simulink model "HvCoorn"  (R2022b)
settings: configuration reference "Icar05FusaMdlCfg" (kept outside this file)
undefined symbols (not defined in the file): BMSActSt_ACChrg, BMSActSt_DCChrg, BMSActSt_disconnect, BMSActSt_offline, BMSActSt_online, BMSActSt_undefined, BMSMainNegRlySt_Clsd_SC, BMSMainNegRlySt_Open_SC, BMSMainNegRlySt_StuckInClsd_SC, BMSMainNegRlySt_StuckInOpen_SC, BMSMainPosRlySt_Clsd_SC, BMSMainPosRlySt_Open_SC, BMSMainPosRlySt_StuckInClsd_SC, BMSPrecRlySt_StuckInOpen_SC, BMSReqSt_ACChrg, BMSReqSt_DCChrg, BMSReqSt_emergencyOffline, BMSReqSt_offline, BMSReqSt_online, Chrg_stCycleBookMod_SC, Chrg_stSingleBookMod_SC, CmpgMod_stInactv_SC, DCDCActSt_buck, DCDCActSt_connected, DCDCActSt_disconnected, DCDCReqSt_buck, DCDCReqSt_standby, EngStrtStop_RefuModDft_SC, EPBActSt_Appld_SC, GearLvr_stDrvGearD_SC, GearLvr_stDrvGearN_SC, GearLvr_stDrvGearP_SC, GearLvr_stDrvGearR_SC, hpp_bACChargeLinkIni_C, hpp_bACChargeLinkOKIni_C, hpp_bAcChgEnaIni_C, hpp_bAcChgPauseIni_C, hpp_bAcLinkTempErrIni_C, hpp_bBattWarmReqIni_C, hpp_bHvilHwErrIni_C, hpp_bHvilStOkIni_C, hpp_bHvRelayClsActIni_C, hpp_bHvRelayOpnActIni_C, hpp_bHvRelayStuckIni_C, hpp_bParked4ChDchgIni_C, hpp_bRemLvBatMntnReqIni_C, hpp_bStartUpReqIni_C, hpp_stHvilCanIni_C, hpp_stWarmTimeCfgRespIni_C, HvCoorn_bAuthEnaSwt_C, HvCoorn_bAuthFailSpdLimOvrd_C, HvCoorn_bAuthFailSpdLimOvrdVal_C, HvCoorn_bAuthStrt_C, HvCoorn_bBMSUnexpdDcnctFailEna_C, HvCoorn_bBuck2RdyBypDCDCEna_C, HvCoorn_bDCChrgFctCfg_C, HvCoorn_bDcChrgWkupEnaChrgLink_C, HvCoorn_bDCDcnct4ACEna_C, HvCoorn_bDCNotBuck2ShtdwnEna_C, HvCoorn_bDrvrLevNotRdyEna_C ... (+295)
libraries: ITKLib x213, simulink x61
(part 8 of 12)

== system HvCoorn/HvCoorn/HVP_HighVoltagePowerOnOffProcedure/A29_V2In ==
  idi_bKeyOn : Inport
  HvCoorn_stHVP : Inport  Port=2
  PwrLimBatt_pwrContnsDChrg : Inport  Port=3
  icbms_pctHVBatSOCDisp : Inport  Port=4
  icobc_stOBCModeV2In : Inport  Port=5
  icobc_stChrgrCnct : Inport  Port=6
  icicm_stIvtrEnaSwt : Inport  Port=7
  ibsw_bCnctElecDvce : Inport  Port=8
  ved_bHvShtdwn : Inport  Port=9
  icobc_stOBCMode : Inport  Port=10
  icobc_stV2LFltTyp : Inport  Port=11
  icicm_bOTAOn : Inport  Port=12
  AND : Logic  Inputs=7  OutDataTypeStr=boolean
  AND1 : Logic  Operator=OR  Inputs=9  OutDataTypeStr=boolean
  AND2 : Logic  OutDataTypeStr=boolean
  AND3 : Logic  OutDataTypeStr=boolean
  AND4 : Logic  OutDataTypeStr=boolean
  AND6 : Logic  Operator=OR  OutDataTypeStr=boolean
  Calibration1 : Constant  Description=[3300]  Value=HvCoorn_pwrBattV2InEnaLowLim_C  SampleTime=-1
      settings: AttributesFormatString=%<Description>
  Calibration2 : Constant  Description=[3300]  Value=HvCoorn_pwrBattV2InExHighLim_C  SampleTime=-1
      settings: AttributesFormatString=%<Description>
  Calibration3 : Constant  Description=[3600]  Value=HvCoorn_tiDiscnctDvceExThd_C  SampleTime=-1
      settings: AttributesFormatString=%<Description>
  Calibration4 : Constant  Description=[1]  Value=HvCoorn_bOTAOnExV2InEna_C  SampleTime=-1
      settings: AttributesFormatString=%<Description>
  Constant10 : Constant  Description=[1]  Value=OBCChrgrCnctnSt_Cnct_SC
      settings: AttributesFormatString=%<Description>
  Constant2 : Constant  Description=[8]  Value=OBCActSt_V2In
      settings: AttributesFormatString=[8]
  Constant3 : Constant  Description=[4]  Value=OBCActSt_V2LAndV2In
      settings: AttributesFormatString=[4]
  Constant4 : Constant  Description=[7]  Value=OBCActSt_failure
      settings: AttributesFormatString=[7]
  Constant5 : Constant  Description=[3]  Value=OBCActSt_charging
      settings: AttributesFormatString=[3]
  Constant6 : Constant  Description=[7]  Value=OBCActSt_failure
      settings: AttributesFormatString=[7]
  Constant9 : Constant  Description=[0]  Value=OBCChrgrCnctnSt_Dcnct_SC
      settings: AttributesFormatString=%<Description>
  EdgeFalling : ITKLib/Memory/EdgeFalling  Tag=initial value = 0
      settings: SourceProductName=ITKC_Lib
  EdgeFalling1 : ITKLib/Memory/EdgeFalling  Tag=initial value = 0
      settings: SourceProductName=ITKC_Lib
  EdgeRising : ITKLib/Memory/EdgeRising  Tag=initial value = 0
      settings: SourceProductName=ITKC_Lib
  Equal{,1,6..11,13..15,17} (12 alike) : RelationalOperator  Operator===  OutDataTypeStr=boolean  RndMeth=Simplest  InputSameDT=off
  Equal12 : RelationalOperator  Operator=<  OutDataTypeStr=boolean  RndMeth=Simplest  InputSameDT=off
  Equal16 : RelationalOperator  Operator=<  OutDataTypeStr=boolean  RndMeth=Simplest  InputSameDT=off
  Equal2 : RelationalOperator  OutDataTypeStr=boolean  RndMeth=Simplest  InputSameDT=off
  Equal3 : RelationalOperator  Operator=>  OutDataTypeStr=boolean  RndMeth=Simplest  InputSameDT=off
  Equal4 : RelationalOperator  Operator=~=  OutDataTypeStr=boolean  RndMeth=Simplest  InputSameDT=off
  Equal5 : RelationalOperator  Operator=~=  OutDataTypeStr=boolean  RndMeth=Simplest  InputSameDT=off
  Not1 : Logic  Operator=NOT  AllPortsSameDT=off  OutDataTypeStr=boolean
  Not6 : Logic  Operator=NOT  AllPortsSameDT=off  OutDataTypeStr=boolean
  OR : Logic  Operator=OR  OutDataTypeStr=boolean
  OR1 : Logic  Operator=OR  OutDataTypeStr=boolean
  OR2 : Logic  Operator=OR  Inputs=3  OutDataTypeStr=boolean
  OR3 : Logic  Operator=OR  Inputs=3  OutDataTypeStr=boolean
  OR7 : Logic  OutDataTypeStr=boolean
  OR8 : Logic  OutDataTypeStr=boolean
  RSLatch : ITKLib/Memory/RSLatch
      settings: SourceProductName=ITKC_Lib
  RSLatch1 : ITKLib/Memory/RSLatch
      settings: SourceProductName=ITKC_Lib
  TaskTime_s2 : Constant  Value=TaskTime_10ms
      settings: AttributesFormatString=[0.01]
  Terminator : Terminator
  TurnOnDelayVari : ITKLib/TimeCounter/TurnOnDelayVari
      settings: AttributesFormatString=TurnOnDelay  SourceProductName=ITKC_Lib
  UnitDelay : UnitDelay  SampleTime=-1  HasFrameUpgradeWarning=on
      settings: AttributesFormatString=<Initial=%<x0>>
  hpp_tiRemHvBatPrecdngSet_C1 : Constant  Description=[20]  Value=HvCoorn_pctHvBatSocV2InExThd_C
      settings: AttributesFormatString=%<Description>
  hpp_tiRemHvBatPrecdngSet_C2 : Constant  Description=[20]  Value=HvCoorn_pctHvBatSocV2InActvThd_C
      settings: AttributesFormatString=%<Description>
  uint1 : Constant  Value=90  OutDataTypeStr=uint8  SampleTime=-1
      settings: AttributesFormatString=%<OutDataTypeStr>
  uint10 : Constant  Value=2  OutDataTypeStr=uint8  SampleTime=-1
      settings: AttributesFormatString=%<OutDataTypeStr>
  uint11 : Constant  Value=3  OutDataTypeStr=uint8  SampleTime=-1
      settings: AttributesFormatString=%<OutDataTypeStr>
  uint2 : Constant  Value=2  OutDataTypeStr=uint8  SampleTime=-1
      settings: AttributesFormatString=%<OutDataTypeStr>
  uint4 : Constant  OutDataTypeStr=uint8  SampleTime=-1
      settings: AttributesFormatString=%<OutDataTypeStr>
  uint8 : Constant  Value=89  OutDataTypeStr=uint8  SampleTime=-1
      settings: AttributesFormatString=%<OutDataTypeStr>
  uint9 : Constant  OutDataTypeStr=uint8  SampleTime=-1
      settings: AttributesFormatString=%<OutDataTypeStr>
  HvCoorn_bV2InReq : Outport  VectorParamsAs1DForOutWhenUnconnected=off
  HvCoorn_bV2InEna : Outport  Port=2  VectorParamsAs1DForOutWhenUnconnected=off
  wires:
  uint8/1 -> Equal/2
  HvCoorn_stHVP/1 -> Equal1/1, Equal/1
  uint1/1 -> Equal1/2
  Equal/1 -> OR/1
  Equal1/1 -> OR/2
  PwrLimBatt_pwrContnsDChrg/1 -> Equal2/1, [PwrLimBatt_pwrContnsDChrg]
  Calibration1/1 -> Equal2/2
  icbms_pctHVBatSOCDisp/1 -> Equal3/1, [icbms_pctHVBatSOCDisp]
  hpp_tiRemHvBatPrecdngSet_C2/1 -> Equal3/2
  [icobc_stOBCMode] -> Equal5/1, Equal4/1
  icobc_stChrgrCnct/1 -> Equal6/1, [icobc_stChrgrCnct]
  Constant9/1 -> Equal6/2
  uint2/1 -> Equal7/2  "Enable"
  icicm_stIvtrEnaSwt/1 -> Equal13/1, Equal7/1
  Equal7/1 -> OR1/1
  ibsw_bCnctElecDvce/1 -> [ibsw_bCnctElecDvce], EdgeRising/1, EdgeFalling1/1, Not1/1
  Equal2/1 -> AND/3
  Equal3/1 -> AND/4
  OR/1 -> AND/1
  idi_bKeyOn/1 -> [idi_bKeyOn], AND/2
  AND/1 -> RSLatch/1  "HvCoorn_bV2InEnaRawSet"
  icobc_stOBCMode/1 -> [icobc_stOBCMode], Equal9/1
  Constant4/1 -> Equal9/2
  [icobc_stChrgrCnct] -> Equal10/1
  Constant10/1 -> Equal10/2
  Calibration2/1 -> Equal12/2
  [PwrLimBatt_pwrContnsDChrg] -> Equal12/1
  Equal12/1 -> AND1/7
  Equal10/1 -> AND1/5
  Equal9/1 -> AND1/4
  Equal16/1 -> AND1/3
  ved_bHvShtdwn/1 -> AND1/2
  OR3/1 -> AND1/1
  uint4/1 -> Equal13/2  "Disable"
  Equal13/1 -> OR3/1
  AND1/1 -> RSLatch/2  "HvCoorn_bV2InEnaRawRst"
  RSLatch/1 -> UnitDelay/1, HvCoorn_bV2InReq/1, OR7/1
  Constant2/1 -> Equal17/2
  [icobc_stOBCMode] -> Equal17/1
  OR7/1 -> HvCoorn_bV2InEna/1
  Equal6/1 -> AND/6
  OR1/1 -> AND/7
  [icbms_pctHVBatSOCDisp] -> Equal16/1
  hpp_tiRemHvBatPrecdngSet_C1/1 -> Equal16/2
  [idi_bKeyOn] -> EdgeFalling/1
  EdgeFalling/1 -> AND1/6
  TaskTime_s2/1 -> TurnOnDelayVari/2
  Calibration3/1 -> TurnOnDelayVari/3
  TurnOnDelayVari/1 -> OR3/3
  Equal8/1 -> AND6/2
  [icobc_stOBCMode] -> Equal8/1
  Constant3/1 -> Equal8/2
  Equal17/1 -> AND6/1
  AND6/1 -> OR7/2
  OR8/1 -> AND/5
  icobc_stOBCModeV2In/1 -> Terminator/1
  Equal4/1 -> OR8/1
  Equal5/1 -> OR8/2
  Constant5/1 -> Equal4/2
  Constant6/1 -> Equal5/2
  EdgeRising/1 -> OR1/2
  UnitDelay/1 -> [HvCoorn_bV2InReqOld]
  Not1/1 -> AND2/1
  [HvCoorn_bV2InReqOld] -> AND2/2
  AND2/1 -> TurnOnDelayVari/1
  [HvCoorn_bV2InReqOld] -> AND3/2
  AND3/1 -> OR3/2
  EdgeFalling1/1 -> AND3/1
  uint10/1 -> Equal11/2
  icobc_stV2LFltTyp/1 -> Equal11/1, Equal14/1, Equal15/1
  uint9/1 -> Equal15/2
  uint11/1 -> Equal14/2
  [ibsw_bCnctElecDvce] -> Not6/1
  Not6/1 -> RSLatch1/2
  Equal14/1 -> OR2/3
  Equal11/1 -> OR2/2
  Equal15/1 -> OR2/1
  OR2/1 -> RSLatch1/1
  RSLatch1/1 -> AND1/9
  AND4/1 -> AND1/8
  icicm_bOTAOn/1 -> AND4/1
  Calibration4/1 -> AND4/2

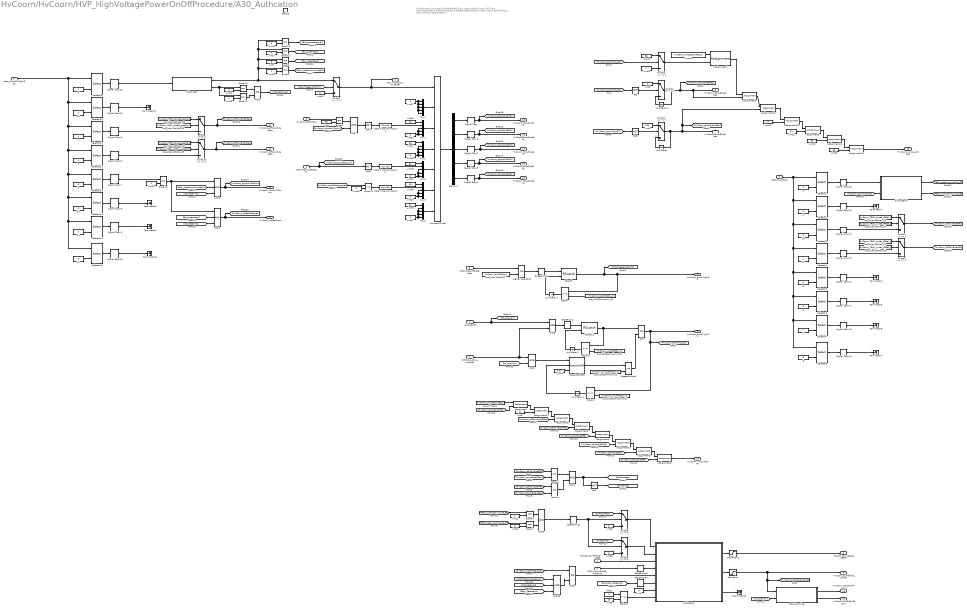
== system HvCoorn/HvCoorn/HVP_HighVoltagePowerOnOffProcedure/A30_Authcation ==
  note: 指令类型
      | 0000无效:0
      | 0001平台网络连接通讯丢失:1
      | 0010防盗校验:2
      | 0011密钥下发:3
      | 0100异常次数清除:4
      | 0101异常次数同步:5
      |
      | 接收模块
      | 0000全部ECU:0
      | 0001仅VCU:1
      | 0010仅BMS:2
      | 0011仅RMCU:3
      | 0100仅TBOX:4
  VCU_E2_counterfaieldEER : Inport
  idi_bKeyOn : Inport  Port=2
  VCCM_flg_Allow_Antitheft : Inport  Port=3
  VCCM_flg_Antitheft_Overtime : Inport  Port=4
  VCCM_flg_Antitheft_Start : Inport  Port=5
  ictcp_noAuthChlgOnReq : Inport  Port=6
  ictcp_noAuthSts : Inport  Port=7
  HvCoorn_stHVPOld : Inport  Port=8
  VCCM_flg_SK_Recep_ok : Inport  Port=9
  Enable : EnablePort
  1 : Constant  Value=3  OutDataTypeStr=single
  10 : Constant  Value=3  OutDataTypeStr=single
  11 : Constant  Value=4  OutDataTypeStr=single
  12 : Constant  Value=5  OutDataTypeStr=single
  13 : Constant  Value=6  OutDataTypeStr=single
  14 : Constant  Value=7  OutDataTypeStr=single
  15 : Constant  Value=8  OutDataTypeStr=single
  16 : Constant  Value=2  OutDataTypeStr=single
  2 : Constant  Value=4  OutDataTypeStr=single
  3 : Constant  Value=5  OutDataTypeStr=single
  4 : Constant  OutDataTypeStr=single
  5 : Constant  OutDataTypeStr=single
  6 : Constant  Value=6  OutDataTypeStr=single
  7 : Constant  Value=7  OutDataTypeStr=single
  8 : Constant  Value=8  OutDataTypeStr=single
  9 : Constant  Value=2  OutDataTypeStr=single
  AND{1,5..8} (5 alike) : Logic  OutDataTypeStr=boolean
  AND10 : Logic  Inputs=3  OutDataTypeStr=boolean
  AND2 : Logic  Operator=OR  OutDataTypeStr=boolean
  AND3 : Logic  Inputs=3  OutDataTypeStr=boolean
  AND4 : Logic  Inputs=3  OutDataTypeStr=boolean
  AND9 : Logic  Operator=OR  OutDataTypeStr=boolean
  Assignment : Assignment  DiagnosticForDimensions=Warning  IndexOptions=Index vector (dialog)  Indices=1  OutputSizes=1
  Assignment1 : Assignment  DiagnosticForDimensions=Warning  IndexOptions=Index vector (dialog)  Indices=6  OutputSizes=1
  Assignment10 : Assignment  DiagnosticForDimensions=Warning  IndexOptions=Index vector (dialog)  Indices=4  OutputSizes=1
  Assignment11 : Assignment  DiagnosticForDimensions=Warning  IndexOptions=Index vector (dialog)  Indices=5  OutputSizes=1
  Assignment12 : Assignment  DiagnosticForDimensions=Warning  IndexOptions=Index vector (dialog)  Indices=7  OutputSizes=1
  Assignment13 : Assignment  DiagnosticForDimensions=Warning  IndexOptions=Index vector (dialog)  Indices=8  OutputSizes=1
  Assignment14 : Assignment  DiagnosticForDimensions=Warning  IndexOptions=Index vector (dialog)  Indices=2  OutputSizes=1
  Assignment2 : Assignment  DiagnosticForDimensions=Warning  IndexOptions=Index vector (dialog)  Indices=3  OutputSizes=1
  Assignment3 : Assignment  DiagnosticForDimensions=Warning  IndexOptions=Index vector (dialog)  Indices=4  OutputSizes=1
  Assignment4 : Assignment  DiagnosticForDimensions=Warning  IndexOptions=Index vector (dialog)  Indices=5  OutputSizes=1
  Assignment5 : Assignment  DiagnosticForDimensions=Warning  IndexOptions=Index vector (dialog)  Indices=7  OutputSizes=1
  Assignment6 : Assignment  DiagnosticForDimensions=Warning  IndexOptions=Index vector (dialog)  Indices=8  OutputSizes=1
  Assignment7 : Assignment  DiagnosticForDimensions=Warning  IndexOptions=Index vector (dialog)  Indices=1  OutputSizes=1
  Assignment8 : Assignment  DiagnosticForDimensions=Warning  IndexOptions=Index vector (dialog)  Indices=6  OutputSizes=1
  Assignment9 : Assignment  DiagnosticForDimensions=Warning  IndexOptions=Index vector (dialog)  Indices=3  OutputSizes=1
  Auth_status : Stateflow chart  TreatAsAtomicUnit=on
  B01_Warnning : Subsystem
  Data Type Conversion : DataTypeConversion  SaturateOnIntegerOverflow=off  RndMeth=Floor
  Data Type Conversion1 : DataTypeConversion  SaturateOnIntegerOverflow=off  RndMeth=Floor
  Data Type Conversion2 : DataTypeConversion  SaturateOnIntegerOverflow=off  RndMeth=Floor
  Delay : Delay  DelayLengthSource=Input port  DelayLengthUpperLimit=200
      settings: InputPortMap=u0,p1
  Delay1 : Delay  DelayLengthSource=Input port  DelayLengthUpperLimit=200
      settings: InputPortMap=u0,p1
  Delay2 : Delay  DelayLengthSource=Input port  DelayLengthUpperLimit=200
      settings: InputPortMap=u0,p1
  Delay3 : Delay  DelayLengthSource=Input port
      settings: InputPortMap=u0,p1
  Demux1 : Demux  Outputs=5
  EdgeRising{,1..4} (5 alike) : ITKLib/Memory/EdgeRising  Tag=initial value = 0
      settings: SourceProductName=ITKC_Lib
  Equal{1..2,6..8,10..13,15} (10 alike) : RelationalOperator  Operator===  OutDataTypeStr=boolean  RndMeth=Simplest  InputSameDT=off
  Equal14 : RelationalOperator  Operator=~=  OutDataTypeStr=boolean  RndMeth=Simplest  InputSameDT=off
  Equal3 : RelationalOperator  Operator===  OutDataTypeStr=boolean
  Equal4 : RelationalOperator  Operator===  OutDataTypeStr=boolean
  GreaterOrEqual : RelationalOperator  OutDataTypeStr=boolean
  Logical Operator6 : Logic  Operator=OR  AllPortsSameDT=off  OutDataTypeStr=boolean
  Multiport Switch : MultiPortSwitch  DataPortOrder=Zero-based contiguous  Inputs=6  zeroidx=on  SaturateOnIntegerOverflow=off  InputSameDT=off
  Mux{1..6} (6 alike) : Mux  Inputs=5
  Not{1..5} (5 alike) : Logic  Operator=NOT  AllPortsSameDT=off  OutDataTypeStr=boolean
  OR2 : Logic  Operator=OR  OutDataTypeStr=boolean
  RSLatch : ITKLib/Memory/RSLatch
      settings: SourceProductName=ITKC_Lib
  RSLatch1 : ITKLib/Memory/RSLatch
      settings: SourceProductName=ITKC_Lib
  Saturation : Saturate  UpperLimit=15  LowerLimit=0
  Saturation1 : Saturate  UpperLimit=15  LowerLimit=0
  Selector{1..16} (16 alike) : Selector  NumberOfDimensions=2  InputPortWidth=10  IndexOptions=Index vector (dialog),Index vector (port)  Indices=1,2  OutputSizes=1,1
  Signal Copy{,1..20} (21 alike) : SignalConversion  OverrideOpt=off
  StopWatchRE1 : ITKLib/TimeCounter/StopWatchRE  Description=""
      settings: SourceProductName=ITKC_Lib
  Subsystem : Subsystem
  Subsystem1 : Subsystem
  Switch{1..4,7..10} (8 alike) : Switch  Criteria=u2 ~= 0  SaturateOnIntegerOverflow=off  InputSameDT=off
      settings: AttributesFormatString=Criteria : %<Criteria>
  Switch5 : Switch  Criteria=u2 ~= 0  OutDataTypeStr=boolean  SaturateOnIntegerOverflow=off  InputSameDT=off
      settings: AttributesFormatString=Criteria : %<Criteria>
  Switch6 : Switch  Criteria=u2 ~= 0  OutDataTypeStr=boolean  SaturateOnIntegerOverflow=off  InputSameDT=off
      settings: AttributesFormatString=Criteria : %<Criteria>
  TRUE : Constant  Description=TRUE  OutDataTypeStr=boolean  SampleTime=-1
      settings: AttributesFormatString=%<Description>
  Terminator{1,4..10,12..13} (10 alike) : Terminator
  Unit Delay{,1..4} (5 alike) : UnitDelay  SampleTime=-1  HasFrameUpgradeWarning=on
      settings: AttributesFormatString=<initial=%<x0>>
  sup_bKeyStrtMan_C : Constant  Description=[0]  Value=HvCoorn_bAuthStrt_C
      settings: AttributesFormatString=%<Description>
  sup_bKeyStrtMan_C1 : Constant  Description=[0]  Value=HvCoorn_TBOX_byte4_FBSet_C
      settings: AttributesFormatString=%<Description>
  sup_bKeyStrtMan_C2 : Constant  Description=[0]  Value=HvCoorn_TBOX_byte4_FBCal_C
      settings: AttributesFormatString=%<Description>
  sup_bKeyStrtMan_C3 : Constant  Description=[0]  Value=HvCoorn_TBOX_byte5_FBCal_C
      settings: AttributesFormatString=%<Description>
  sup_bKeyStrtMan_C4 : Constant  Description=[0]  Value=HvCoorn_TBOX_byte5_FBSet_C
      settings: AttributesFormatString=%<Description>
  sup_bKeyStrtMan_C5 : Constant  Description=[0]  Value=HvCoorn_TBOX_byte5_reqCal_C
      settings: AttributesFormatString=%<Description>
  sup_bKeyStrtMan_C6 : Constant  Description=[0]  Value=HvCoorn_TBOX_byte5_reqSet_C
      settings: AttributesFormatString=%<Description>
  sup_bKeyStrtMan_C7 : Constant  Description=[0]  Value=HvCoorn_TBOX_byte4_reqCal_C
      settings: AttributesFormatString=%<Description>
  sup_bKeyStrtMan_C8 : Constant  Description=[0]  Value=HvCoorn_TBOX_byte4_reqSet_C
      settings: AttributesFormatString=%<Description>
  sup_tiChgConndown_C : Constant  Description=[1800]  Value=HvCoorn_tiAuthStartDly_C
      settings: AttributesFormatString=%<Description>
  sup_tiChgConndown_C1 : Constant  Description=[200]  Value=HvCoorn_nAuthRstDly_C
      settings: AttributesFormatString=%<Description>
  sup_tiChgConndown_C2 : Constant  Description=[200]  Value=HvCoorn_nAuthRstDly_C
      settings: AttributesFormatString=%<Description>
  sup_tiChgConndown_C3 : Constant  Description=[200]  Value=HvCoorn_nAuthRstDly_C
      settings: AttributesFormatString=%<Description>
  sup_uThres_C : Constant  Description="[0  0  0  0  0  0  0  0]"  Value=HvCoorn_uVCU2tboxFB_C  OutDataTypeStr=uint8
      settings: AttributesFormatString=%<Description>
  uint{1,15,24,29,31..35,37,40} (11 alike) : Constant  Value=0  OutDataTypeStr=uint8  SampleTime=-1
      settings: AttributesFormatString=%<OutDataTypeStr>
  uint{6,11,25..26,28} (5 alike) : Constant  OutDataTypeStr=uint8  SampleTime=-1
      settings: AttributesFormatString=%<OutDataTypeStr>
  uint12 : Constant  Value=2  OutDataTypeStr=uint8  SampleTime=-1
      settings: AttributesFormatString=%<OutDataTypeStr>
  uint13 : Constant  Value=17  OutDataTypeStr=uint8  SampleTime=-1
      settings: AttributesFormatString=%<OutDataTypeStr>
  uint2 : Constant  Value=17  OutDataTypeStr=uint8  SampleTime=-1
      settings: AttributesFormatString=%<OutDataTypeStr>
  uint21 : Constant  Value=34  OutDataTypeStr=uint8  SampleTime=-1
      settings: AttributesFormatString=%<OutDataTypeStr>
  uint22 : Constant  Value=51  OutDataTypeStr=uint8  SampleTime=-1
      settings: AttributesFormatString=%<OutDataTypeStr>
  uint23 : Constant  Value=68  OutDataTypeStr=uint8  SampleTime=-1
      settings: AttributesFormatString=%<OutDataTypeStr>
  uint27 : Constant  Value=4  OutDataTypeStr=uint8  SampleTime=-1
      settings: AttributesFormatString=%<OutDataTypeStr>
  uint3 : Constant  Value=100  OutDataTypeStr=uint8  SampleTime=-1
      settings: AttributesFormatString=%<OutDataTypeStr>
  uint36 : Constant  Value=20  OutDataTypeStr=uint8  SampleTime=-1
      settings: AttributesFormatString=%<OutDataTypeStr>
  uint38 : Constant  Value=0  OutDataTypeStr=boolean  SampleTime=-1
      settings: AttributesFormatString=%<OutDataTypeStr>
  uint39 : Constant  Value=0  OutDataTypeStr=boolean  SampleTime=-1
      settings: AttributesFormatString=%<OutDataTypeStr>
  uint4 : Constant  Description=SystemReadyWait  Value=89  OutDataTypeStr=uint8
      settings: AttributesFormatString=|
      | %<OutDataTypeStr>
      | %<Description>
  uint41 : Constant  Value=5  OutDataTypeStr=uint8  SampleTime=-1
      settings: AttributesFormatString=%<OutDataTypeStr>
  uint43 : Constant  Value=36  OutDataTypeStr=uint8  SampleTime=-1
      settings: AttributesFormatString=%<OutDataTypeStr>
  uint44 : Constant  Value=0.01  OutDataTypeStr=single  SampleTime=-1
      settings: AttributesFormatString=%<OutDataTypeStr>
  uint46 : Constant  Description="[0  0  0  0  0  0  0  0]"  Value=HvCoorn_uVCU2tboxReq_C  OutDataTypeStr=uint8  SampleTime=-1
      settings: AttributesFormatString=%<Description>
  uint47 : Constant  Value=36  OutDataTypeStr=uint8  SampleTime=-1
      settings: AttributesFormatString=%<OutDataTypeStr>
  uint48 : Constant  Value=52  OutDataTypeStr=uint8  SampleTime=-1
      settings: AttributesFormatString=%<OutDataTypeStr>
  uint49 : Constant  Value=68  OutDataTypeStr=uint8  SampleTime=-1
      settings: AttributesFormatString=%<OutDataTypeStr>
  uint5 : Constant  Value=10  OutDataTypeStr=uint8  SampleTime=-1
      settings: AttributesFormatString=%<OutDataTypeStr>
  uint50 : Constant  Value=84  OutDataTypeStr=uint8  SampleTime=-1
      settings: AttributesFormatString=%<OutDataTypeStr>
  uint7 : Constant  Value=3  OutDataTypeStr=uint8  SampleTime=-1
      settings: AttributesFormatString=%<OutDataTypeStr>
  VCU_Instruction_Type_FB : Outport  VectorParamsAs1DForOutWhenUnconnected=off
  HvCoorn_bAntiTrig430 : Outport  Port=2  VectorParamsAs1DForOutWhenUnconnected=off
  HvCoorn_bAntiTrig42C : Outport  Port=3  VectorParamsAs1DForOutWhenUnconnected=off
  VCU_E2_counterfaieldEEW : Outport  Port=4  VectorParamsAs1DForOutWhenUnconnected=off
  HvCoorn_authfailed_conter : Outport  Port=5  VectorParamsAs1DForOutWhenUnconnected=off
  HvCoorn_stVcuByte5Req : Outport  Port=6  VectorParamsAs1DForOutWhenUnconnected=off
  HvCoorn_stVcuByte4Req : Outport  Port=7  VectorParamsAs1DForOutWhenUnconnected=off
  HvCoorn_bAuthHvStrtLim : Outport  Port=8  VectorParamsAs1DForOutWhenUnconnected=off
  HvCoorn_bClearZero : Outport  Port=9  VectorParamsAs1DForOutWhenUnconnected=off
  HvCoorn_stAuthChkFailLvl : Outport  Port=10  VectorParamsAs1DForOutWhenUnconnected=off
  HvCoorn_stTboxByte5Req : Outport  Port=11  VectorParamsAs1DForOutWhenUnconnected=off
  HvCoorn_stTboxByte4Req : Outport  Port=12  VectorParamsAs1DForOutWhenUnconnected=off
  HvCoorn_stVcuByte3Fb : Outport  Port=13  VectorParamsAs1DForOutWhenUnconnected=off
  HvCoorn_stVcuByte2Fb : Outport  Port=14  VectorParamsAs1DForOutWhenUnconnected=off
  HvCoorn_stVcuByte1Fb : Outport  Port=15  VectorParamsAs1DForOutWhenUnconnected=off
  HvCoorn_stVcuByte0Fb : Outport  Port=16  VectorParamsAs1DForOutWhenUnconnected=off
  HvCoorn_noVcuAuthFb : Outport  Port=17  VectorParamsAs1DForOutWhenUnconnected=off
  HvCoorn_noVcuAuthReq : Outport  Port=18  VectorParamsAs1DForOutWhenUnconnected=off
  HvCoorn_stVcuByte7Fb : Outport  Port=19  VectorParamsAs1DForOutWhenUnconnected=off
  " HvCoorn_bAuthFailSpdLim" : Outport  Port=20  VectorParamsAs1DForOutWhenUnconnected=off
  wires:
  RSLatch/1 -> Delay/1, HvCoorn_bAntiTrig430/1, [VCU_Trigger_430_TX]
  [HvCoorn_bAntiTrig42C] -> Switch3/2
  uint43/1 -> Switch3/1
  uint15/1 -> Switch3/3
  Switch5/1 -> Auth_status/1(authsuccess)  "authsuccess"
  Saturation/1 -> HvCoorn_authfailed_conter/1, B01_Warnning/1(HvCoorn_authfailed_conter), [HvCoorn_authfailed_conter]  "HvCoorn_authfailed_conter"
  VCU_E2_counterfaieldEER/1 -> Auth_status/3(authfailed_n_conterEER)
  Auth_status/2(authfailed_n_conter) -> Saturation/1
  Auth_status/1(authfailed_n_conterEEW) -> Saturation1/1
  AND6/1 -> StopWatchRE1/1
  uint44/1 -> StopWatchRE1/3
  sup_tiChgConndown_C/1 -> GreaterOrEqual/2
  StopWatchRE1/1 -> GreaterOrEqual/1
  GreaterOrEqual/1 -> OR2/2
  Subsystem/2(TBOX_receiver_module_req) -> Equal10/1, Equal11/1
  Switch7/1 -> VCU_Instruction_Type_FB/1, Multiport Switch/1  "VCU_Instruction_Type_FB"
  [HvCoorn_stTboxByte5Fb] -> Equal3/1
  [HvCoorn_stTboxByte4Fb] -> Equal4/1
  AND1/1 -> [authsuccess], Not1/1
  Equal3/1 -> AND1/1
  [HvCoorn_stVcuByte5Req] -> Equal3/2
  [HvCoorn_stVcuByte4Req] -> Equal4/2
  Equal4/1 -> AND1/2
  Not1/1 -> [authfailed]
  uint3/1 -> Switch1/1
  Unit Delay/1 -> Switch1/3
  Unit Delay1/1 -> Switch2/3
  [HvCoorn_bAntiTrig42C] -> Not2/1
  Not2/1 -> Switch2/2
  Not3/1 -> Switch1/2
  [HvCoorn_bAntiTrig42C] -> Not3/1
  [TBOX_Instruction_Type_FB] -> Equal6/1
  uint11/1 -> Equal6/2
  uint12/1 -> Equal7/2
  [TBOX_receiver_module_FB] -> Equal7/1
  uint21/1 -> Assignment8/2
  uint22/1 -> Assignment12/2
  Equal10/1 -> AND2/1
  uint24/1 -> Equal10/2
  uint25/1 -> Equal11/2
  Equal11/1 -> AND2/2
  AND2/1 -> [VCU_receiver]
  Equal8/1 -> [tbox_lostcoummunication]
  uint26/1 -> Equal8/2
  uint27/1 -> Equal12/2
  Equal12/1 -> [fault_clearzero]
  Equal13/1 -> AND3/1, AND4/1
  uint28/1 -> Equal13/2
  [tbox_lostcoummunication] -> AND3/2
  [VCU_receiver] -> AND3/3
  AND3/1 -> HvCoorn_bAuthHvStrtLim/1, [HvCoorn_bAuthHvStrtLim]  "HvCoorn_bAuthHvStrtLim"
  [VCU_receiver] -> AND4/3
  [fault_clearzero] -> AND4/2
  B01_Warnning/1(HvCoorn_stAuthChkFailLvl) -> HvCoorn_stAuthChkFailLvl/1
  uint1/1 -> Auth_status/7(TCP_AnomalyOfAntitheftCheck)
  uint37/1 -> Mux4/5, Mux4/4, Mux4/3, Mux4/2, Mux4/1
  uint34/1 -> Mux1/3, Mux1/4, Mux1/5
  uint35/1 -> Mux2/2, Mux2/3, Mux2/4, Mux2/5
  Mux4/1 -> Multiport Switch/2
  Mux2/1 -> Multiport Switch/4
  uint29/1 -> Mux5/5, Mux5/4, Mux5/3
  Mux1/1 -> Multiport Switch/3
  Mux6/1 -> Multiport Switch/5
  uint31/1 -> Mux6/3, Mux6/4, Mux6/5
  Mux5/1 -> Multiport Switch/6
  Mux3/1 -> Multiport Switch/7
  uint33/1 -> Equal14/2
  Equal14/1 -> Data Type Conversion/1
  [HvCoorn_authfailed_conter] -> Equal14/1
  uint36/1 -> Mux1/1
  Multiport Switch/1 -> Demux1/1
  Demux1/2 -> Signal Copy1/1
  Demux1/4 -> Signal Copy3/1
  Demux1/5 -> Signal Copy4/1
  VCCM_flg_Antitheft_Overtime/1 -> EdgeRising3/1
  Equal6/1 -> AND5/1
  Equal7/1 -> AND5/2
  uint39/1 -> Switch5/3
  [authsuccess] -> Switch5/1
  AND5/1 -> EdgeRising1/1  "HvCoorn_flg_Authtrigger"
  uint38/1 -> Switch6/3
  [authfailed] -> Switch6/1
  EdgeRising1/1 -> Switch6/2, Switch5/2
  uint6/1 -> Switch2/1
  EdgeRising2/1 -> RSLatch/1
  Delay/1 -> Unit Delay2/1
  sup_tiChgConndown_C2/1 -> Delay/2
  [VCU_Trigger_430_TX] -> Switch7/2
  uint40/1 -> Switch7/3
  [HvCoorn_bClearZeropre] -> AND9/1
  Equal15/1 -> [fault_counterequal]
  uint41/1 -> Equal15/2
  [idi_bKeyOn] -> AND6/2
  [fault_counterequal] -> EdgeRising4/1
  Unit Delay2/1 -> RSLatch/2
  Unit Delay4/1 -> StopWatchRE1/2
  EdgeRising3/1 -> Auth_status/4(VCCM_flg_Antitheft_Overtime)
  sup_uThres_C/1 -> Assignment/1
  Assignment2/1 -> Assignment3/1
  [HvCoorn_stVcuByte7Fb] -> Assignment/2
  [HvCoorn_stTboxByte5Req] -> Assignment2/2
  [HvCoorn_stTboxByte4Req] -> Assignment3/2
  Assignment3/1 -> Assignment4/1
  [HvCoorn_stVcuByte3Fb] -> Assignment4/2
  Assignment4/1 -> Assignment1/1
  Assignment14/1 -> Assignment2/1
  Assignment1/1 -> Assignment5/1
  Assignment5/1 -> Assignment6/1
  Assignment6/1 -> HvCoorn_noVcuAuthFb/1
  Assignment13/1 -> HvCoorn_noVcuAuthReq/1
  Assignment12/1 -> Assignment13/1
  Assignment8/1 -> Assignment12/1
  Assignment7/1 -> Assignment9/1
  Assignment11/1 -> Assignment8/1
  uint13/1 -> Assignment11/2
  Assignment10/1 -> Assignment11/1
  Switch1/1 -> [HvCoorn_stVcuByte4Req], Assignment10/2, HvCoorn_stVcuByte4Req/1, Unit Delay/1  "HvCoorn_stVcuByte4Req"
  Switch2/1 -> Assignment9/2, HvCoorn_stVcuByte5Req/1, [HvCoorn_stVcuByte5Req], Unit Delay1/1  "HvCoorn_stVcuByte5Req"
  Assignment9/1 -> Assignment10/1
  uint46/1 -> Assignment7/1
  7/1 -> Selector7/2
  10/1 -> Selector3/2
  Selector5/1 -> Signal Copy12/1
  12/1 -> Selector5/2
  8/1 -> Selector8/2
  Selector6/1 -> Signal Copy17/1
  Selector7/1 -> Signal Copy18/1
  Selector3/1 -> Signal Copy14/1
  Selector8/1 -> Signal Copy19/1
  Selector2/1 -> Signal Copy15/1
  5/1 -> Selector1/2
  6/1 -> Selector6/2
  Selector4/1 -> Signal Copy13/1
  Selector1/1 -> Signal Copy16/1
  9/1 -> Selector2/2
  ictcp_noAuthSts/1 -> Selector7/1, Selector8/1, Selector6/1, Selector5/1, Selector4/1, Selector3/1, Selector2/1, Selector1/1
  11/1 -> Selector4/2
  EdgeRising4/1 -> Auth_status/6(fault_counterequal)
  uint23/1 -> Assignment13/2
  Demux1/3 -> Signal Copy2/1
  [HvCoorn_stVcuByte0Fb] -> Assignment6/2
  [HvCoorn_stVcuByte1Fb] -> Assignment5/2
  [HvCoorn_stVcuByte2Fb] -> Assignment1/2
  Demux1/1 -> Signal Copy/1
  uint32/1 -> Mux3/2, Mux3/3, Mux3/4, Mux3/5
  Switch6/1 -> Auth_status/2(authfailed)  "authfailed"
  Saturation1/1 -> VCU_E2_counterfaieldEEW/1
  sup_tiChgConndown_C1/1 -> Delay1/2
  Delay1/1 -> Unit Delay4/1
  OR2/1 -> HvCoorn_bAntiTrig42C/1, Delay1/1, [HvCoorn_bAntiTrig42C]
  uint47/1 -> Mux2/1
  uint48/1 -> Mux6/1
  Data Type Conversion/1 -> Mux5/2
  uint49/1 -> Mux5/1
  uint50/1 -> Mux3/1
  B01_Warnning/2(HvCoorn_bAuthFailSpdLim) -> " HvCoorn_bAuthFailSpdLim"/1
  Signal Copy/1 -> HvCoorn_stVcuByte7Fb/1, [HvCoorn_stVcuByte7Fb]  "HvCoorn_stVcuByte7Fb"
  Signal Copy1/1 -> HvCoorn_stVcuByte3Fb/1, [HvCoorn_stVcuByte3Fb]  "HvCoorn_stVcuByte3Fb"
  Signal Copy2/1 -> HvCoorn_stVcuByte2Fb/1, [HvCoorn_stVcuByte2Fb]  "HvCoorn_stVcuByte2Fb"
  Signal Copy3/1 -> [HvCoorn_stVcuByte1Fb], HvCoorn_stVcuByte1Fb/1  "HvCoorn_stVcuByte1Fb"
  Signal Copy4/1 -> HvCoorn_stVcuByte0Fb/1, [HvCoorn_stVcuByte0Fb]  "HvCoorn_stVcuByte0Fb"
  1/1 -> Selector11/2
  13/1 -> Selector14/2
  16/1 -> Selector10/2
  Selector9/1 -> Signal Copy20/1
  Selector13/1 -> Signal Copy7/1
  4/1 -> Selector9/2
  14/1 -> Selector15/2
  Selector16/1 -> Signal Copy10/1
  Selector15/1 -> Signal Copy9/1
  Selector14/1 -> Signal Copy8/1
  15/1 -> Selector16/2
  2/1 -> Selector12/2
  Selector11/1 -> Signal Copy5/1
  Selector10/1 -> Signal Copy11/1
  3/1 -> Selector13/2
  Selector12/1 -> Signal Copy6/1
  Switch9/1 -> HvCoorn_stTboxByte5Req/1, [HvCoorn_stTboxByte5Req]  "HvCoorn_stTboxByte5Req"
  Switch10/1 -> HvCoorn_stTboxByte4Req/1, [HvCoorn_stTboxByte4Req]  "HvCoorn_stTboxByte4Req"
  Signal Copy7/1 -> Equal13/1  "HvCoorn_stTboxByte3Req"
  Signal Copy8/1 -> Terminator8/1  "HvCoorn_stTboxByte2Req"
  Signal Copy9/1 -> Terminator9/1  "HvCoorn_stTboxByte1Req"
  Signal Copy10/1 -> Terminator10/1  "HvCoorn_stTboxByte0Req"
  Signal Copy11/1 -> Terminator12/1  "HvCoorn_stTboxByte6Req"
  Signal Copy12/1 -> Terminator4/1  "HvCoorn_stTboxByte3Fb"
  Switch8/1 -> [HvCoorn_stTboxByte4Fb]  "HvCoorn_stTboxByte4Fb"
  Switch4/1 -> [HvCoorn_stTboxByte5Fb]  "HvCoorn_stTboxByte5Fb"
  Signal Copy15/1 -> Terminator1/1  "HvCoorn_stTboxByte6Fb"
  Signal Copy16/1 -> Subsystem1/1(HvCoorn_stTboxByte7Fb)  "HvCoorn_stTboxByte7Fb"
  Signal Copy17/1 -> Terminator5/1  "HvCoorn_stTboxByte2Fb"
  Signal Copy18/1 -> Terminator6/1  "HvCoorn_stTboxByte1Fb"
  Signal Copy19/1 -> Terminator7/1  "HvCoorn_stTboxByte0Fb"
  Switch3/1 -> Assignment7/2  "HvCoorn_stVcuByte7Req"
  Signal Copy20/1 -> Subsystem/1(HvCoorn_stTboxByte7Req)  "HvCoorn_stTboxByte7Req"
  Subsystem1/1(TBOX_receiver_module_FB) -> [TBOX_receiver_module_FB]
  Subsystem1/2(TBOX_Instruction_Type_FB) -> [TBOX_Instruction_Type_FB]
  ictcp_noAuthChlgOnReq/1 -> Selector15/1, Selector16/1, Selector14/1, Selector13/1, Selector12/1, Selector11/1, Selector10/1, Selector9/1
  [idi_bKeyOn] -> B01_Warnning/2(idi_bKeyOn)
  AND4/1 -> HvCoorn_bClearZero/1, [HvCoorn_bClearZeropre]  "HvCoorn_bClearZero"
  HvCoorn_stHVPOld/1 -> Equal1/1
  uint4/1 -> Equal1/2
  Equal1/1 -> AND7/1
  [HvCoorn_bAuthHvStrtLim] -> AND7/2
  AND7/1 -> Not4/1
  Not4/1 -> Data Type Conversion1/1
  sup_bKeyStrtMan_C/1 -> Logical Operator6/2
  VCCM_flg_Antitheft_Start/1 -> Logical Operator6/1
  Logical Operator6/1 -> EdgeRising2/1
  EdgeRising/1 -> RSLatch1/1
  Unit Delay3/1 -> RSLatch1/2
  sup_tiChgConndown_C3/1 -> Delay2/2
  Delay2/1 -> Unit Delay3/1
  RSLatch1/1 -> OR2/1, Delay2/1
  Data Type Conversion1/1 -> Mux1/2
  VCCM_flg_Allow_Antitheft/1 -> AND8/2, AND6/1
  AND8/1 -> EdgeRising/1
  Assignment/1 -> Assignment14/1
  uint2/1 -> Assignment14/2
  Signal Copy14/1 -> Switch4/3
  Signal Copy13/1 -> Switch8/3
  sup_bKeyStrtMan_C1/1 -> Switch8/2
  sup_bKeyStrtMan_C2/1 -> Switch8/1
  sup_bKeyStrtMan_C4/1 -> Switch4/2
  sup_bKeyStrtMan_C3/1 -> Switch4/1
  sup_bKeyStrtMan_C5/1 -> Switch9/1
  sup_bKeyStrtMan_C6/1 -> Switch9/2
  Signal Copy5/1 -> Switch9/3
  Signal Copy6/1 -> Switch10/3
  sup_bKeyStrtMan_C8/1 -> Switch10/2
  sup_bKeyStrtMan_C7/1 -> Switch10/1
  VCCM_flg_SK_Recep_ok/1 -> Not5/1, [VCCM_flg_SK_Recep_ok]
  Not5/1 -> Data Type Conversion2/1
  [HvCoorn_bAntiTrig42C] -> Subsystem1/2(VCU_Trigger_42C_TX)
  Data Type Conversion2/1 -> Mux6/2
  Auth_status/3(auth_enum) -> Terminator13/1  "auth_enum"
  uint5/1 -> Delay3/2
  Delay3/1 -> Auth_status/8(Hvcoorn_bEEReadOver)
  TRUE/1 -> Delay3/1
  idi_bKeyOn/1 -> AND8/1, [idi_bKeyOn]
  AND9/1 -> Auth_status/5(HvCoorn_bClearZero)
  Subsystem/1(TBOX_Instruction_Type_req) -> Equal2/1, Equal12/1, Equal15/1, Equal8/1, Switch7/1
  uint7/1 -> Equal2/2
  Equal2/1 -> [tbox_Seektrans]
  AND10/1 -> AND9/2
  [VCU_receiver] -> AND10/2
  [tbox_Seektrans] -> AND10/3
  [VCCM_flg_SK_Recep_ok] -> AND10/1

== system HvCoorn/HvCoorn/HVP_HighVoltagePowerOnOffProcedure/A30_ISGNotRdy ==
  HvCoorn_bStartUpReq : Inport
  icems_stEng : Inport  Port=2
  HvCoorn_stHVPOld : Inport  Port=3
  icems_nAct : Inport  Port=4
  AND1 : Logic  OutDataTypeStr=boolean
  Calibration1 : Constant  Description=[1]  Value=HvCoorn_tiISGNoRdyNoStrtReqDly_C  SampleTime=-1
      settings: AttributesFormatString=%<Description>
  Calibration2 : Constant  Description=[50]  Value=HvCoorn_nHvDownEngSpdMaxThd_C  SampleTime=-1
      settings: AttributesFormatString=%<Description>
  Calibration3 : Constant  Description=[0.1]  Value=HvCoorn_tiEngSpdHvDownAllwThd_C  SampleTime=-1
      settings: AttributesFormatString=%<Description>
  Lower : RelationalOperator  Operator=<  OutDataTypeStr=boolean
  Not : Logic  Operator=NOT  AllPortsSameDT=off  OutDataTypeStr=boolean
  OR : Logic  Operator=OR  Inputs=3  OutDataTypeStr=boolean
  OR1 : Logic  OutDataTypeStr=boolean
  Relational Operator3 : RelationalOperator  Operator=~=  OutDataTypeStr=boolean
      settings: DeleteFcn=if exist('delete_tlblock','file')==2,delete_tlblock(gcbh);end  NameChangeFcn=if exist('rename_tlblock','file')==2,rename_tlblock(gcbh);end  OpenFcn=if exist('tl_open_blockdlg','file')==2,tl_open_blockdlg(gcbh);else,open_system(gcbh,'parameter');end
  Relational Operator4 : RelationalOperator  Operator=~=  OutDataTypeStr=boolean
      settings: DeleteFcn=if exist('delete_tlblock','file')==2,delete_tlblock(gcbh);end  NameChangeFcn=if exist('rename_tlblock','file')==2,rename_tlblock(gcbh);end  OpenFcn=if exist('tl_open_blockdlg','file')==2,tl_open_blockdlg(gcbh);else,open_system(gcbh,'parameter');end
  Relational Operator6 : RelationalOperator  Operator=~=  OutDataTypeStr=boolean
      settings: DeleteFcn=if exist('delete_tlblock','file')==2,delete_tlblock(gcbh);end  NameChangeFcn=if exist('rename_tlblock','file')==2,rename_tlblock(gcbh);end  OpenFcn=if exist('tl_open_blockdlg','file')==2,tl_open_blockdlg(gcbh);else,open_system(gcbh,'parameter');end
  TaskTime_s1 : Constant  Value=TaskTime_10ms
      settings: AttributesFormatString=[0.01]
  TaskTime_s3 : Constant  Value=TaskTime_10ms
      settings: AttributesFormatString=[0.01]
  TurnOnDelayVari1 : ITKLib/TimeCounter/TurnOnDelayVari
      settings: AttributesFormatString=TurnOnDelay  SourceProductName=ITKC_Lib
  TurnOnDelayVari2 : ITKLib/TimeCounter/TurnOnDelayVari
      settings: AttributesFormatString=TurnOnDelay  SourceProductName=ITKC_Lib
  icemsSt_Run_SC2 : Constant  Description=[3]  Value=icems_stEngRun_SC  OutDataTypeStr=Inherit: Inherit via back propagation  SampleTime=-1
      settings: AttributesFormatString=%<Description>  CopyFcn=if exist('tl_reset_reviewflag','file')==2,tl_reset_reviewflag(gcbh);end  DeleteFcn=if exist('delete_tlblock','file')==2,delete_tlblock(gcbh);end  NameChangeFcn=if exist('rename_tlblock','file')==2,rename_tlblock(gcbh);end  OpenFcn=if exist('tl_open_blockdlg','file')==2,tl_open_blockdlg(gcbh);else,open_system(gcbh,'parameter');end
  uint1 : Constant  Value=90  OutDataTypeStr=uint8  SampleTime=-1
      settings: AttributesFormatString=%<OutDataTypeStr>
  uint8 : Constant  Value=89  OutDataTypeStr=uint8  SampleTime=-1
      settings: AttributesFormatString=%<OutDataTypeStr>
  HvCoorn_bAPUNotRdy : Outport  VectorParamsAs1DForOutWhenUnconnected=off
  wires:
  TaskTime_s3/1 -> TurnOnDelayVari1/2
  Calibration1/1 -> TurnOnDelayVari1/3
  HvCoorn_bStartUpReq/1 -> Not/1
  Not/1 -> TurnOnDelayVari1/1
  TurnOnDelayVari1/1 -> OR/1
  icems_stEng/1 -> Relational Operator6/1
  icemsSt_Run_SC2/1 -> Relational Operator6/2
  Relational Operator6/1 -> OR1/1
  HvCoorn_stHVPOld/1 -> Relational Operator4/1, Relational Operator3/1
  uint8/1 -> Relational Operator3/2
  uint1/1 -> Relational Operator4/2
  Relational Operator3/1 -> AND1/1
  Relational Operator4/1 -> AND1/2
  AND1/1 -> OR/3
  OR/1 -> HvCoorn_bAPUNotRdy/1  "HvCoorn_bAPUNotRdy"
  Lower/1 -> OR1/2
  icems_nAct/1 -> Lower/1
  Calibration2/1 -> Lower/2
  Calibration3/1 -> TurnOnDelayVari2/3
  TaskTime_s1/1 -> TurnOnDelayVari2/2
  OR1/1 -> TurnOnDelayVari2/1
  TurnOnDelayVari2/1 -> OR/2

== system HvCoorn/HvCoorn/HVP_HighVoltagePowerOnOffProcedure/A31_VoltModReq ==
  EngStrtStop_bHVPRdy : Inport
  ipf_bPCAN0x130Vld : Inport  Port=2
  DTC_bBMSFltLvl6 : Inport  Port=3
  DTC_bBMSFltLvl7 : Inport  Port=4
  DTC_bBMSFltLvl8 : Inport  Port=5
  HvCoorn_stVoltModOld : Inport  Port=6
  EngStrtStop_bEngStrtAllw : Inport  Port=7
  HybCoorn_bEngStrtFail : Inport  Port=8
  icems_stEng : Inport  Port=9
  ved_bInhbEngStrt : Inport  Port=10
  icems_nAct : Inport  Port=11
  icbms_stMainPosRly : Inport  Port=12
  icbms_stMainNegRly : Inport  Port=13
  icbms_iHVBat : Inport  Port=14
  icfm_uAct : Inport  Port=15
  icdc_uHvAct : Inport  Port=16
  icisg_uAct : Inport  Port=17
  icisg_stMod : Inport  Port=18
  DTC_bBMSFltLvl5 : Inport  Port=19
  HvCoorn_bStartUpReq : Inport  Port=20
  HvCoorn_stHVP : Inport  Port=21
  BrkPedDev_bBrk : Inport  Port=22
  GearLvr_stDrvGear : Inport  Port=23
  VehSpd_vVeh : Inport  Port=24
  icfm_stMode : Inport  Port=25
  icrm_stMode : Inport  Port=26
  icdc_stMode : Inport  Port=27
  VehCfg_bFrntMotByp : Inport  Port=28
  HvGrid_pwrLoadAct : Inport  Port=29
  icrm_uAct : Inport  Port=30
  Subsystem : Subsystem
  Subsystem1 : Subsystem
  Subsystem2 : Subsystem
  Subsystem3 : Subsystem
  Subsystem4 : Subsystem
  HvCoorn_bDft2EngStrt : Outport  VectorParamsAs1DForOutWhenUnconnected=off
  HvCoorn_bEngStrt2HvDisb : Outport  Port=2  VectorParamsAs1DForOutWhenUnconnected=off
  HvCoorn_bHvDisb2HvDcnct : Outport  Port=3  VectorParamsAs1DForOutWhenUnconnected=off
  HvCoorn_bHvDcnct2HvReq : Outport  Port=4  VectorParamsAs1DForOutWhenUnconnected=off
  HvCoorn_bHvReq2VoltModRdy : Outport  Port=5  VectorParamsAs1DForOutWhenUnconnected=off
  HvCoorn_bEngStrt2Dft : Outport  Port=6  VectorParamsAs1DForOutWhenUnconnected=off
  HvCoorn_bHvDisb2Dft : Outport  Port=7  VectorParamsAs1DForOutWhenUnconnected=off
  HvCoorn_bHvDcnct2Dft : Outport  Port=8  VectorParamsAs1DForOutWhenUnconnected=off
  HvCoorn_bHvReq2Dft : Outport  Port=9  VectorParamsAs1DForOutWhenUnconnected=off
  HvCoorn_bVoltModRdy2Dft : Outport  Port=10  VectorParamsAs1DForOutWhenUnconnected=off
  HvCoorn_bHvInit2Dft : Outport  Port=11  VectorParamsAs1DForOutWhenUnconnected=off
  HvCoorn_bHvCnt2Dft : Outport  Port=12  VectorParamsAs1DForOutWhenUnconnected=off
  HvCoorn_bDCBuck2Dft : Outport  Port=13  VectorParamsAs1DForOutWhenUnconnected=off
  HvCoorn_bHvDcnct2HvInit : Outport  Port=14  VectorParamsAs1DForOutWhenUnconnected=off
  HvCoorn_bHvInit2HvCnt : Outport  Port=15  VectorParamsAs1DForOutWhenUnconnected=off
  HvCoorn_bHvCnt2DCBuck : Outport  Port=16  VectorParamsAs1DForOutWhenUnconnected=off
  HvCoorn_bHvInit2EngStrt : Outport  Port=17  VectorParamsAs1DForOutWhenUnconnected=off
  HvCoorn_bHvCnt2EngStrt : Outport  Port=18  VectorParamsAs1DForOutWhenUnconnected=off
  HvCoorn_bDCBuck2EngStrt : Outport  Port=19  VectorParamsAs1DForOutWhenUnconnected=off
  HvCoorn_bVoltModHvDisbOvtiErr : Outport  Port=20  VectorParamsAs1DForOutWhenUnconnected=off
  HvCoorn_bVoltModHvDcnctOvtiErr : Outport  Port=21  VectorParamsAs1DForOutWhenUnconnected=off
  HvCoorn_bVoltModHvReqOvtiErr : Outport  Port=22  VectorParamsAs1DForOutWhenUnconnected=off
  HvCoorn_bDft2EngStrtRaw : Outport  Port=23  VectorParamsAs1DForOutWhenUnconnected=off
  wires:
  EngStrtStop_bHVPRdy/1 -> Subsystem/1(EngStrtStop_bHVPRdy)
  ipf_bPCAN0x130Vld/1 -> Subsystem/2(ipf_bPCAN0x130Vld)
  DTC_bBMSFltLvl6/1 -> Subsystem/3(DTC_bBMSFltLvl6)
  DTC_bBMSFltLvl7/1 -> Subsystem/4(DTC_bBMSFltLvl7)
  DTC_bBMSFltLvl8/1 -> Subsystem/5(DTC_bBMSFltLvl8)
  EngStrtStop_bEngStrtAllw/1 -> Subsystem/6(EngStrtStop_bEngStrtAllw)
  HybCoorn_bEngStrtFail/1 -> Subsystem/7(HybCoorn_bEngStrtFail)
  HvCoorn_stVoltModOld/1 -> [HvCoorn_stVoltModOld], Subsystem/8(HvCoorn_stVoltModOld)
  Subsystem/4(HvCoorn_bDft2EngStrt) -> HvCoorn_bDft2EngStrt/1
  Subsystem1/1(HvCoorn_bEngStrt2HvDisb) -> HvCoorn_bEngStrt2HvDisb/1
  Subsystem2/1(HvCoorn_bHvDisb2HvDcnct) -> HvCoorn_bHvDisb2HvDcnct/1
  Subsystem2/2(HvCoorn_bHvDcnct2HvReq) -> HvCoorn_bHvDcnct2HvReq/1
  Subsystem3/1(HvCoorn_bHvReq2VoltModRdy) -> HvCoorn_bHvReq2VoltModRdy/1
  icems_stEng/1 -> Subsystem1/1(icems_stEng)
  icems_nAct/1 -> Subsystem1/3(icems_nAct)
  ved_bInhbEngStrt/1 -> Subsystem1/2(ved_bInhbEngStrt)
  icbms_stMainPosRly/1 -> Subsystem2/1(icbms_stMainPosRly)
  icbms_stMainNegRly/1 -> Subsystem2/2(icbms_stMainNegRly)
  icbms_iHVBat/1 -> Subsystem2/3(icbms_iHVBat)
  icfm_uAct/1 -> [icfm_uAct], Subsystem3/1(icfm_uAct)
  icisg_uAct/1 -> Subsystem3/3(icisg_uAct)
  icisg_stMod/1 -> [icisg_stMod], Subsystem3/4(icisg_stMod)
  Subsystem/1(HvCoorn_bVoltModHvDisbOvtiErr) -> HvCoorn_bVoltModHvDisbOvtiErr/1
  Subsystem/2(HvCoorn_bVoltModHvDcnctOvtiErr) -> HvCoorn_bVoltModHvDcnctOvtiErr/1
  Subsystem/3(HvCoorn_bVoltModHvReqOvtiErr) -> HvCoorn_bVoltModHvReqOvtiErr/1
  DTC_bBMSFltLvl5/1 -> Subsystem/9(DTC_bBMSFltLvl5)
  Subsystem/5(HvCoorn_bEngStrt2Dft) -> HvCoorn_bEngStrt2Dft/1
  Subsystem/6(HvCoorn_bHvDisb2Dft) -> HvCoorn_bHvDisb2Dft/1
  Subsystem/16(HvCoorn_bBMSFltRcvGearPN) -> [HvCoorn_bBMSFltRcvGearPN]
  Subsystem/7(HvCoorn_bHvDcnct2Dft) -> HvCoorn_bHvDcnct2Dft/1
  Subsystem/8(HvCoorn_bHvReq2Dft) -> HvCoorn_bHvReq2Dft/1
  Subsystem/9(HvCoorn_bVoltModRdy2Dft) -> HvCoorn_bVoltModRdy2Dft/1
  Subsystem/10(HvCoorn_bHvInit2Dft) -> HvCoorn_bHvInit2Dft/1
  Subsystem/11(HvCoorn_bHvCnt2Dft) -> HvCoorn_bHvCnt2Dft/1
  Subsystem/12(HvCoorn_bDCBuck2Dft) -> HvCoorn_bDCBuck2Dft/1
  Subsystem/13(HvCoorn_bHvInit2EngStrt) -> HvCoorn_bHvInit2EngStrt/1
  Subsystem/14(HvCoorn_bHvCnt2EngStrt) -> HvCoorn_bHvCnt2EngStrt/1
  Subsystem/15(HvCoorn_bDCBuck2EngStrt) -> HvCoorn_bDCBuck2EngStrt/1
  HvCoorn_bStartUpReq/1 -> [HvCoorn_bStartUpReq], Subsystem/10(HvCoorn_bStartUpReq)
  HvCoorn_stHVP/1 -> [HvCoorn_stHVP], Subsystem/11(HvCoorn_stHVP)
  BrkPedDev_bBrk/1 -> Subsystem/12(BrkPedDev_bBrk)
  GearLvr_stDrvGear/1 -> Subsystem/13(GearLvr_stDrvGear)
  VehSpd_vVeh/1 -> Subsystem/14(VehSpd_vVeh)
  Subsystem4/1(HvCoorn_bHvDcnct2HvInit) -> HvCoorn_bHvDcnct2HvInit/1
  Subsystem4/2(HvCoorn_bHvInit2HvCnt) -> HvCoorn_bHvInit2HvCnt/1
  Subsystem4/3(HvCoorn_bHvCnt2DCBuck) -> HvCoorn_bHvCnt2DCBuck/1
  [HvCoorn_bStartUpReq] -> Subsystem4/1(HvCoorn_bStartUpReq)
  [HvCoorn_stHVP] -> Subsystem4/2(HvCoorn_stHVP)
  [HvCoorn_bBMSFltRcvGearPN] -> Subsystem4/3(HvCoorn_bBMSFltRcvGearPN)
  icfm_stMode/1 -> Subsystem4/4(icfm_stMode)
  icrm_stMode/1 -> Subsystem4/5(icrm_stMode)
  icdc_stMode/1 -> Subsystem4/6(icdc_stMode)
  VehCfg_bFrntMotByp/1 -> Subsystem4/8(VehCfg_bFrntMotByp)
  HvGrid_pwrLoadAct/1 -> Subsystem4/9(HvGrid_pwrLoadAct)
  icdc_uHvAct/1 -> Subsystem4/11(icdc_uHvAct)
  icrm_uAct/1 -> [icrm_uAct], Subsystem3/2(icrm_uAct)
  [icisg_stMod] -> Subsystem4/7(icisg_stMod)
  [icfm_uAct] -> Subsystem4/10(icfm_uAct)
  [icrm_uAct] -> Subsystem4/12(icrm_uAct)
  [HvCoorn_stVoltModOld] -> Subsystem2/4(HvCoorn_stVoltModOld)
  Subsystem/17(HvCoorn_bDft2EngStrtRaw) -> HvCoorn_bDft2EngStrtRaw/1

== system HvCoorn/HvCoorn/HVP_HighVoltagePowerOnOffProcedure/A33_ISGVoltReq ==
  icfm_uAct : Inport
  icdc_uHvAct : Inport  Port=2
  icisg_uAct : Inport  Port=3
  HvCoorn_stVoltMod : Inport  Port=4
  Equal1 : RelationalOperator  Operator===  OutDataTypeStr=boolean
  Equal2 : RelationalOperator  Operator===  OutDataTypeStr=boolean
  MinMax : MinMax  Function=max  Inputs=3  SaturateOnIntegerOverflow=on
  OR : Logic  Operator=OR  OutDataTypeStr=boolean
  RampLimiter : ITKLib/Filter/RampLimiter
      settings: SourceProductName=ITKC_Lib
  Switch : Switch  Criteria=u2 ~= 0  SaturateOnIntegerOverflow=off  InputSameDT=off
      settings: AttributesFormatString=Criteria : %<Criteria>
  icbms_undefined1 : Constant  Description=[5]  Value=VoltMod_stVoltModRdy_SC  OutDataTypeStr=uint8
      settings: AttributesFormatString=%<Description>
  icbms_undefined2 : Constant  Description=[4]  Value=VoltMod_stHvReq_SC  OutDataTypeStr=uint8
      settings: AttributesFormatString=%<Description>
  sup_uIpuShutdown_C : Constant  Description=[385]  Value=HvCoorn_uVoltModISGReq_C
      settings: AttributesFormatString=%<Description>
  sup_uIpuShutdown_C1 : Constant  Description=[2]  Value=HvCoorn_duVoltModISGReqIncGrdt_C
      settings: AttributesFormatString=%<Description>
  sup_uIpuShutdown_C2 : Constant  Description=[2]  Value=HvCoorn_duVoltModISGReqDecGrdt_C
      settings: AttributesFormatString=%<Description>
  HvCoorn_uISGReq : Outport
  wires:
  icisg_uAct/1 -> MinMax/3
  icdc_uHvAct/1 -> MinMax/2
  icfm_uAct/1 -> MinMax/1
  RampLimiter/1 -> HvCoorn_uISGReq/1
  MinMax/1 -> Switch/3
  Switch/1 -> RampLimiter/1
  sup_uIpuShutdown_C/1 -> Switch/1
  HvCoorn_stVoltMod/1 -> Equal1/1, Equal2/1
  icbms_undefined2/1 -> Equal1/2
  OR/1 -> Switch/2, RampLimiter/4
  sup_uIpuShutdown_C1/1 -> RampLimiter/2
  sup_uIpuShutdown_C2/1 -> RampLimiter/3
  Equal1/1 -> OR/1
  icbms_undefined1/1 -> Equal2/2
  Equal2/1 -> OR/2

== system HvCoorn/HvCoorn/HVP_HighVoltagePowerOnOffProcedure/Subsystem ==
  VehCfg_stCycCdn : Inport
  AND : Logic  OutDataTypeStr=boolean
  Constant53 : Constant  Description=[0]  Value=VehCfg_stCycCdnWLTC_SC
      settings: AttributesFormatString=%<Description>
  Equal1 : RelationalOperator  Operator===  OutDataTypeStr=boolean
  sup_bEmEnaDCUStMan_C : Constant  Description=[1]  Value=HvCoorn_bAuthEnaSwt_C  OutDataTypeStr=boolean
      settings: AttributesFormatString=%<Description>
  HvCoorn_bAuthEna : Outport
  wires:
  VehCfg_stCycCdn/1 -> Equal1/1
  Constant53/1 -> Equal1/2
  Equal1/1 -> AND/1
  AND/1 -> HvCoorn_bAuthEna/1
  sup_bEmEnaDCUStMan_C/1 -> AND/2
